simulink model "FOC_For_PMSM"  (R2023b)
settings: Solver=VariableStepAuto  StartTime=0.0  StopTime=1  MaxStep=1e-4  RelTol=1e-3
values from neighbouring files (symbols this model uses):
  B = 11e-5    (= 0.00011)    [FOC_For_PMSM.m]    (also in FOC_For_PMSM_Parameters.m)
  Idref = 0    [FOC_For_PMSM.m]    (also in FOC_For_PMSM_Parameters.m)
  J = 0.47e-4    (= 4.7e-05)    [FOC_For_PMSM.m]    (also in FOC_For_PMSM_Parameters.m)
  Kcq = (2*zeta*wn*L) - Rs    (= 84.52)    [FOC_For_PMSM.m]    (also in FOC_For_PMSM_Parameters.m)
  Kcs = ((2*zeta*wns) - (B/J)) / ((1.5 *(p^2)*flux)/J)    (= 0.00768666666667)    [FOC_For_PMSM.m]    (also in FOC_For_PMSM_Parameters.m)
  Ld = 7e-2    (= 0.07)    [FOC_For_PMSM.m]    (also in FOC_For_PMSM_Parameters.m)
  Lq = 7e-2    (= 0.07)    [FOC_For_PMSM.m]    (also in FOC_For_PMSM_Parameters.m)
  p = 2    [FOC_For_PMSM.m]    (also in FOC_For_PMSM_Parameters.m)
  Rs = 2.98    [FOC_For_PMSM.m]    (also in FOC_For_PMSM_Parameters.m)
  speed_ref = 500    [FOC_For_PMSM.m]    (also in FOC_For_PMSM_Parameters.m)
libraries: slpidlib x3, spsDCVoltageSourceLib x1, spsUniversalBridgeLib x1, spsdq0toabcLib x1, spsPermanentMagnetSynchronousMachineLib x1, spsThreePhaseVIMeasurementLib x1, spspowerguiLib x1
settings Model: Creator=Admin  LastModifiedBy=hkurt
settings SolverCC: ZeroCrossAlgorithm=Adaptive
settings DebuggingCC: MaskedZcDiagnostic=none  IgnoredZcDiagnostic=none

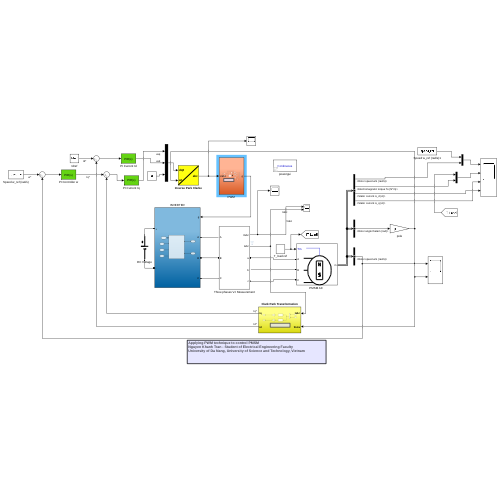
[thumbnail: Simulink's stored preview of the top-level diagram]
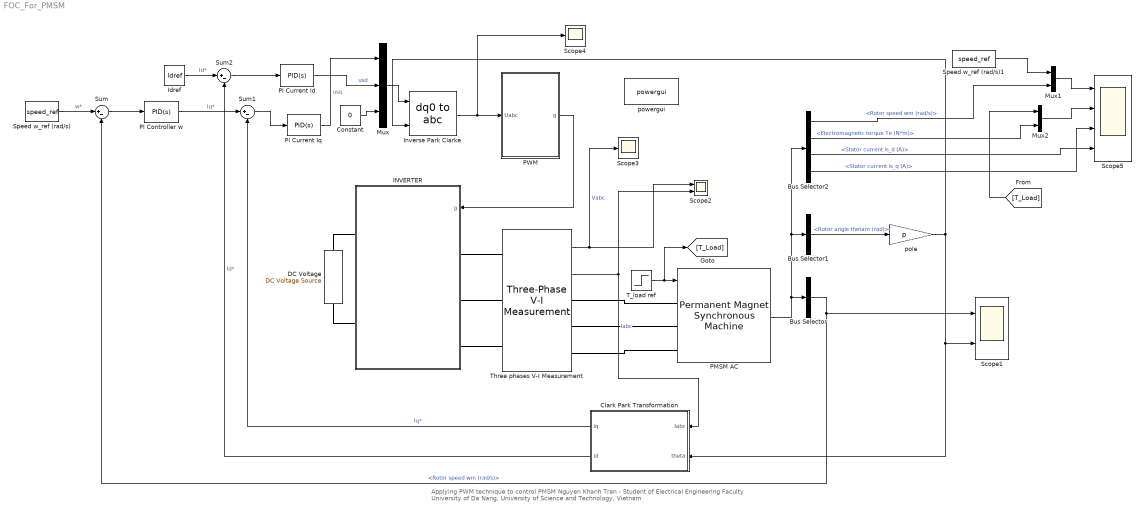
== system FOC_For_PMSM ==
  note: Applying PWM technique to control PMSM
      | Nguyen Khanh Tran - Student of Electrical Engineering Faculty
      | University of Da Nang, University of Science and Technology, Vietnam
  Bus Selector : BusSelector  OutputSignals=Rotor speed wm (rad/s)
  Bus Selector1 : BusSelector  OutputSignals=Rotor angle thetam (rad)
  Bus Selector2 : BusSelector  OutputSignals=Rotor speed wm (rad/s),Electromagnetic torque Te (N*m),Stator current is_d (A),Stator current is_q (A)
  Clark Park Transformation : Subsystem
  Constant : Constant  Value=0
  DC Voltage : spsDCVoltageSourceLib/DC Voltage Source  Amplitude=600  Measurements=None
  INVERTER : Subsystem
  Idref : Constant  Value=Idref
  Inverse Park Clarke : spsdq0toabcLib/dq0 to abc  Alignment=Aligned with phase A axis
  Mux : Mux  Inputs=3
  Mux1 : Mux  Inputs=2
  Mux2 : Mux  Inputs=2
  PI Controller w : slpidlib/PID Controller  Controller=PID  Form=Parallel  TimeDomain=Continuous-time  UseExternalTs=off  SampleTime=-1  IntegratorMethod=Forward Euler  FilterMethod=Forward Euler  ControllerParametersSource=internal  P=Kcs  I=Kcs/0.2001  UseKiTs=off  D=0  N=100  UseFilter=on  TunerSelectOption=Transfer Function Based (PID Tuner App)  InitialConditionSource=internal  InitialConditionForIntegrator=0  InitialConditionForFilter=0  DifferentiatorICPrevScaledInput=0  ExternalReset=none  TrackingMode=off  Kt=1  LimitOutput=off  SatLimitsSource=internal  UpperSaturationLimit=inf  LowerSaturationLimit=-inf  LinearizeAsGain=on  AntiWindupMode=none  Kb=1  LimitIntegrator=off  UpperIntegratorSaturationLimit=inf  LowerIntegratorSaturationLimit=-inf  POutMin=[]  POutMax=[]  IOutMin=[]  IOutMax=[]  DOutMin=[]  DOutMax=[]  NOutMin=[]  NOutMax=[]  SumOutMin=[]  SumOutMax=[]  SaturationOutMin=[]  SaturationOutMax=[]  PParamMin=[]  PParamMax=[]  IParamMin=[]  IParamMax=[]  DParamMin=[]  DParamMax=[]  NParamMin=[]  NParamMax=[]  KbParamMin=[]  KbParamMax=[]  KtParamMin=[]  KtParamMax=[]  KbOutMin=[]  KbOutMax=[]  KtOutMin=[]  KtOutMax=[]  IntegratorOutMin=[]  IntegratorOutMax=[]  FilterOutMin=[]  FilterOutMax=[]  SumI1OutMin=[]  SumI1OutMax=[]  SumI2OutMin=[]  SumI2OutMax=[]  SumI3OutMin=[]  SumI3OutMax=[]  SumI4OutMin=[]  SumI4OutMax=[]  SumDOutMin=[]  SumDOutMax=[]  DifferentiatorOutMin=[]  DifferentiatorOutMax=[]  FilterDiffOutCoefMin=[]  FilterDiffOutCoefMax=[]  ReciprocalOutMin=[]  ReciprocalOutMax=[]  SumDenOutMin=[]  SumDenOutMax=[]  SumNumOutMin=[]  SumNumOutMax=[]  DivideOutMin=[]  DivideOutMax=[]  UdiffTsProdOutMin=[]  UdiffTsProdOutMax=[]  NTsProdOutMin=[]  NTsProdOutMax=[]  UintegralTsProdOutMin=[]  UintegralTsProdOutMax=[]  UngainTsProdOutMin=[]  UngainTsProdOutMax=[]  ClampingZeroOutDataTypeStr=Inherit: Inherit via back propagation  ClampingZeroOutMin=[]  ClampingZeroOutMax=[]  FilterDenConstantOutDataTypeStr=Inherit: Inherit via back propagation  FilterDenConstantOutMin=[]  FilterDenConstantOutMax=[]  PCopyOutDataTypeStr=Inherit: Inherit via back propagation  PCopyOutMin=[]  PCopyOutMax=[]  NCopyOutDataTypeStr=Inherit: Inherit via back propagation  NCopyOutMin=[]  NCopyOutMax=[]  IntegratorContinuousStateAttributes=''  IntegratorStateMustResolveToSignalObject=off  IntegratorRTWStateStorageClass=Auto  FilterContinuousStateAttributes=''  FilterStateMustResolveToSignalObject=off  FilterRTWStateStorageClass=Auto  ParallelPVariant=InternalParameters  IdealPVariant=Disabled  IVariant=InternalParameters  DVariant=InternalParameters  IntegratorVariant=Continuous  SatVariant=Disabled  AWVariant=Passthrough  PCopyVariant=Disabled  TRVariant=Disabled  FdbkBlocksVariant=Forward  IdealPFdbkVariant=Disabled  SatFdbkVariant=Disabled  DerivativeFilterVariant=ContFilter  NVariant=InternalParameters  NCopyVariant=Disabled  FilterICVariant=InternalICsFilter  IntegratorICVariant=InternalICs  ExternalResetVariant=Disabled  TRSumVariant=Passthrough  SumFdbkVariant=Disabled  SumVariant=Sum_PID  TsampFilterVariant=InternalTs  TsampNgainVariant=Passthrough  TsampIntegralVariant=Disabled_SignalSpec  ExternalSaturationOutDataTypeStr=Inherit: Same as second input
  PI Current Id : slpidlib/PID Controller  Controller=PID  Form=Parallel  TimeDomain=Continuous-time  UseExternalTs=off  SampleTime=-1  IntegratorMethod=Forward Euler  FilterMethod=Forward Euler  ControllerParametersSource=internal  P=Kcq  I=Kcq/0.001  UseKiTs=off  D=0  N=100  UseFilter=on  TunerSelectOption=Transfer Function Based (PID Tuner App)  InitialConditionSource=internal  InitialConditionForIntegrator=0  InitialConditionForFilter=0  DifferentiatorICPrevScaledInput=0  ExternalReset=none  TrackingMode=off  Kt=1  LimitOutput=off  SatLimitsSource=internal  UpperSaturationLimit=inf  LowerSaturationLimit=-inf  LinearizeAsGain=on  AntiWindupMode=none  Kb=1  LimitIntegrator=off  UpperIntegratorSaturationLimit=inf  LowerIntegratorSaturationLimit=-inf  POutMin=[]  POutMax=[]  IOutMin=[]  IOutMax=[]  DOutMin=[]  DOutMax=[]  NOutMin=[]  NOutMax=[]  SumOutMin=[]  SumOutMax=[]  SaturationOutMin=[]  SaturationOutMax=[]  PParamMin=[]  PParamMax=[]  IParamMin=[]  IParamMax=[]  DParamMin=[]  DParamMax=[]  NParamMin=[]  NParamMax=[]  KbParamMin=[]  KbParamMax=[]  KtParamMin=[]  KtParamMax=[]  KbOutMin=[]  KbOutMax=[]  KtOutMin=[]  KtOutMax=[]  IntegratorOutMin=[]  IntegratorOutMax=[]  FilterOutMin=[]  FilterOutMax=[]  SumI1OutMin=[]  SumI1OutMax=[]  SumI2OutMin=[]  SumI2OutMax=[]  SumI3OutMin=[]  SumI3OutMax=[]  SumI4OutMin=[]  SumI4OutMax=[]  SumDOutMin=[]  SumDOutMax=[]  DifferentiatorOutMin=[]  DifferentiatorOutMax=[]  FilterDiffOutCoefMin=[]  FilterDiffOutCoefMax=[]  ReciprocalOutMin=[]  ReciprocalOutMax=[]  SumDenOutMin=[]  SumDenOutMax=[]  SumNumOutMin=[]  SumNumOutMax=[]  DivideOutMin=[]  DivideOutMax=[]  UdiffTsProdOutMin=[]  UdiffTsProdOutMax=[]  NTsProdOutMin=[]  NTsProdOutMax=[]  UintegralTsProdOutMin=[]  UintegralTsProdOutMax=[]  UngainTsProdOutMin=[]  UngainTsProdOutMax=[]  ClampingZeroOutDataTypeStr=Inherit: Inherit via back propagation  ClampingZeroOutMin=[]  ClampingZeroOutMax=[]  FilterDenConstantOutDataTypeStr=Inherit: Inherit via back propagation  FilterDenConstantOutMin=[]  FilterDenConstantOutMax=[]  PCopyOutDataTypeStr=Inherit: Inherit via back propagation  PCopyOutMin=[]  PCopyOutMax=[]  NCopyOutDataTypeStr=Inherit: Inherit via back propagation  NCopyOutMin=[]  NCopyOutMax=[]  IntegratorContinuousStateAttributes=''  IntegratorStateMustResolveToSignalObject=off  IntegratorRTWStateStorageClass=Auto  FilterContinuousStateAttributes=''  FilterStateMustResolveToSignalObject=off  FilterRTWStateStorageClass=Auto  ParallelPVariant=InternalParameters  IdealPVariant=Disabled  IVariant=InternalParameters  DVariant=InternalParameters  IntegratorVariant=Continuous  SatVariant=Disabled  AWVariant=Passthrough  PCopyVariant=Disabled  TRVariant=Disabled  FdbkBlocksVariant=Forward  IdealPFdbkVariant=Disabled  SatFdbkVariant=Disabled  DerivativeFilterVariant=ContFilter  NVariant=InternalParameters  NCopyVariant=Disabled  FilterICVariant=InternalICsFilter  IntegratorICVariant=InternalICs  ExternalResetVariant=Disabled  TRSumVariant=Passthrough  SumFdbkVariant=Disabled  SumVariant=Sum_PID  TsampFilterVariant=InternalTs  TsampNgainVariant=Passthrough  TsampIntegralVariant=Disabled_SignalSpec  ExternalSaturationOutDataTypeStr=Inherit: Same as second input
  PI Current Iq : slpidlib/PID Controller  Controller=PID  Form=Parallel  TimeDomain=Continuous-time  UseExternalTs=off  SampleTime=-1  IntegratorMethod=Forward Euler  FilterMethod=Forward Euler  ControllerParametersSource=internal  P=Kcq  I=Kcq/0.001  UseKiTs=off  D=0  N=100  UseFilter=on  TunerSelectOption=Transfer Function Based (PID Tuner App)  InitialConditionSource=internal  InitialConditionForIntegrator=0  InitialConditionForFilter=0  DifferentiatorICPrevScaledInput=0  ExternalReset=none  TrackingMode=off  Kt=1  LimitOutput=off  SatLimitsSource=internal  UpperSaturationLimit=inf  LowerSaturationLimit=-inf  LinearizeAsGain=on  AntiWindupMode=none  Kb=1  LimitIntegrator=off  UpperIntegratorSaturationLimit=inf  LowerIntegratorSaturationLimit=-inf  POutMin=[]  POutMax=[]  IOutMin=[]  IOutMax=[]  DOutMin=[]  DOutMax=[]  NOutMin=[]  NOutMax=[]  SumOutMin=[]  SumOutMax=[]  SaturationOutMin=[]  SaturationOutMax=[]  PParamMin=[]  PParamMax=[]  IParamMin=[]  IParamMax=[]  DParamMin=[]  DParamMax=[]  NParamMin=[]  NParamMax=[]  KbParamMin=[]  KbParamMax=[]  KtParamMin=[]  KtParamMax=[]  KbOutMin=[]  KbOutMax=[]  KtOutMin=[]  KtOutMax=[]  IntegratorOutMin=[]  IntegratorOutMax=[]  FilterOutMin=[]  FilterOutMax=[]  SumI1OutMin=[]  SumI1OutMax=[]  SumI2OutMin=[]  SumI2OutMax=[]  SumI3OutMin=[]  SumI3OutMax=[]  SumI4OutMin=[]  SumI4OutMax=[]  SumDOutMin=[]  SumDOutMax=[]  DifferentiatorOutMin=[]  DifferentiatorOutMax=[]  FilterDiffOutCoefMin=[]  FilterDiffOutCoefMax=[]  ReciprocalOutMin=[]  ReciprocalOutMax=[]  SumDenOutMin=[]  SumDenOutMax=[]  SumNumOutMin=[]  SumNumOutMax=[]  DivideOutMin=[]  DivideOutMax=[]  UdiffTsProdOutMin=[]  UdiffTsProdOutMax=[]  NTsProdOutMin=[]  NTsProdOutMax=[]  UintegralTsProdOutMin=[]  UintegralTsProdOutMax=[]  UngainTsProdOutMin=[]  UngainTsProdOutMax=[]  ClampingZeroOutDataTypeStr=Inherit: Inherit via back propagation  ClampingZeroOutMin=[]  ClampingZeroOutMax=[]  FilterDenConstantOutDataTypeStr=Inherit: Inherit via back propagation  FilterDenConstantOutMin=[]  FilterDenConstantOutMax=[]  PCopyOutDataTypeStr=Inherit: Inherit via back propagation  PCopyOutMin=[]  PCopyOutMax=[]  NCopyOutDataTypeStr=Inherit: Inherit via back propagation  NCopyOutMin=[]  NCopyOutMax=[]  IntegratorContinuousStateAttributes=''  IntegratorStateMustResolveToSignalObject=off  IntegratorRTWStateStorageClass=Auto  FilterContinuousStateAttributes=''  FilterStateMustResolveToSignalObject=off  FilterRTWStateStorageClass=Auto  ParallelPVariant=InternalParameters  IdealPVariant=Disabled  IVariant=InternalParameters  DVariant=InternalParameters  IntegratorVariant=Continuous  SatVariant=Disabled  AWVariant=Passthrough  PCopyVariant=Disabled  TRVariant=Disabled  FdbkBlocksVariant=Forward  IdealPFdbkVariant=Disabled  SatFdbkVariant=Disabled  DerivativeFilterVariant=ContFilter  NVariant=InternalParameters  NCopyVariant=Disabled  FilterICVariant=InternalICsFilter  IntegratorICVariant=InternalICs  ExternalResetVariant=Disabled  TRSumVariant=Passthrough  SumFdbkVariant=Disabled  SumVariant=Sum_PID  TsampFilterVariant=InternalTs  TsampNgainVariant=Passthrough  TsampIntegralVariant=Disabled_SignalSpec  ExternalSaturationOutDataTypeStr=Inherit: Same as second input
  "PMSM AC  " : spsPermanentMagnetSynchronousMachineLib/Permanent Magnet Synchronous Machine  NbPhases=3  FluxDistribution=Sinusoidal  RotorType=Salient-pole  MechanicalLoad=Torque Tm  PresetModel=No  ShowDetailedParameters=on  MeasurementBus=off  Resistance=Rs  Inductance=8.5e-3  dqInductances=[Ld, Lq]  La=0.000395  MachineConstant=Flux linkage established by magnets (V.s)  Flux=flux  VoltageCst=45.345  TorqueCst=0.375  Flat=120  Mechanical=[J B p 0]  PolePairs=4  InitialConditions=[0,0, 0,0]  InitialConditions5ph=[0 0 0 0 0 0]  RefAngle=90 degrees behind phase A axis (modified Park)  IterativeDiscreteModel=Trapezoidal non iterative  TsBlock=-1  TsPowergui=0
  "PWM " : Subsystem
  Scope1 : Scope  NumInputPorts=2
  Scope2 : Scope  NumInputPorts=2
  Scope3 : Scope
  Scope4 : Scope
  Scope5 : Scope  NumInputPorts=4
  Speed w_ref (rad/s) : Constant  Value=speed_ref
  Speed w_ref (rad/s)1 : Constant  Value=speed_ref
  Sum : Sum  Inputs=|+-
  Sum1 : Sum  Inputs=|+-
  Sum2 : Sum  Inputs=|+-
  T_load ref : Step  Time=0.3  SampleTime=0
  Three phases V-I Measurement : spsThreePhaseVIMeasurementLib/Three-Phase V-I Measurement  VoltageMeasurement=phase-to-phase  SetLabelV=off  LabelV=Vabc  Vpu=off  VpuLL=off  CurrentMeasurement=yes  SetLabelI=off  LabelI=Iabc  Ipu=off  Pbase=100e6  Vbase=500e3  OutputType=Complex  PhasorSimulation=off  PSBequivalent=0
  pole : Gain  Gain=p
  powergui : spspowerguiLib/powergui  Priority=1  SimulationMode=Continuous  SampleTime=50e-6  frequency=60  Iterations=50  frequencyindice=0  Pbase=100e6  ErrMax=1e-4  UnitsV=kV  UnitsW=MW  buscounter=0  FunctionMessages=off  echomessages=off  EnableUseOfTLC=off  CurrentSourceSwitches=off  DisableSnubberDevices=off  DisableRonSwitches=off  DisableVfSwitches=off  DisplayEquations=off  AutomaticDiscreteSolvers=off  SolverType=Tustin/Backward Euler (TBE)  Interpol=off  ExternalGateDelay=off  methode=off  Ts=100  x0status=blocks  SPID=on  SwTol=0  HookPort=off  NonlinearTolerance=1e-4  nMaxIteration=100  ContinueOnMaxIteration=off  RestoreLinks=warning  ResistiveCurrentMeasurement=off  Frange=[0:2:500]  Ylog=off  Xlog=on  ShowGrid=off  save=off  variable=ZData  structure=0  ZoomFFT=off  StartTime=0.0  cycles=1  DisplayStyle=1  fundamental=60  FreqAxis=off  MaxFrequency=1000  frequencyindicesteady=1  RmsSteady=1  display=off
  wires:
  Sum/1 -> PI Controller w/1
  Speed w_ref (rad/s)/1 -> Sum/1  "w*"
  "PMSM AC  "/1 -> Bus Selector2/1, Bus Selector1/1, Bus Selector/1
  Bus Selector1/1 -> pole/1  "<Rotor angle thetam (rad)>"
  Bus Selector2/2 -> Mux2/2  "<Electromagnetic torque Te (N*m)>"
  Bus Selector2/3 -> Scope5/4  "<Stator current is_d (A)>"
  Bus Selector2/4 -> Scope5/3  "<Stator current is_q (A)>"
  Three phases V-I Measurement/1 -> Scope3/1, Scope2/1  "Vabc"
  Sum1/1 -> PI Current Iq/1
  Sum2/1 -> PI Current Id/1
  Idref/1 -> Sum2/1  "Id*"
  PI Controller w/1 -> Sum1/1  "Iq*"
  "PWM "/1(g) -> INVERTER/1(g)
  Three phases V-I Measurement/2 -> Clark Park Transformation/1(Iabc), Scope2/2  "Iabc"
  Mux/1 -> Inverse Park Clarke/1
  Inverse Park Clarke/1 -> Scope4/1, "PWM "/1(Uabc)
  Constant/1 -> Mux/3
  pole/1 -> Clark Park Transformation/2(theta), Scope1/2, Inverse Park Clarke/2
  PI Current Id/1 -> Mux/2  "usd"
  PI Current Iq/1 -> Mux/1  "usq"
  Bus Selector/1 -> Sum/2, Scope1/1  "<Rotor speed wm (rad/s)>"
  Clark Park Transformation/1(iq) -> Sum1/2  "Iq*"
  Clark Park Transformation/2(id) -> Sum2/2  "Id*"
  [T_Load] -> Mux2/1
  Speed w_ref (rad/s)1/1 -> Mux1/1
  Mux1/1 -> Scope5/1
  Mux2/1 -> Scope5/2
  Bus Selector2/1 -> Mux1/2  "<Rotor speed wm (rad/s)>"
  T_load ref/1 -> [T_Load], "PMSM AC  "/1
  connections:
  INVERTER/LConn1 -- Three phases V-I Measurement/LConn1
  INVERTER/LConn2 -- Three phases V-I Measurement/LConn2
  INVERTER/LConn3 -- Three phases V-I Measurement/LConn3
  Three phases V-I Measurement/RConn1 -- "PMSM AC  "/LConn1
  Three phases V-I Measurement/RConn2 -- "PMSM AC  "/LConn2
  Three phases V-I Measurement/RConn3 -- "PMSM AC  "/LConn3
  DC Voltage/RConn1 -- INVERTER/RConn1
  INVERTER/RConn2 -- DC Voltage/LConn1

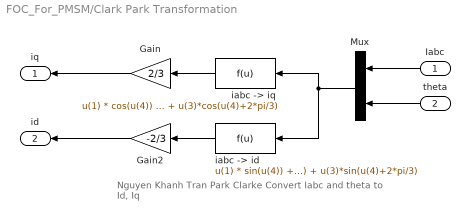
== system FOC_For_PMSM/Clark Park Transformation ==
  note: Nguyen Khanh Tran
      | Park Clarke
      | Convert Iabc and theta to Id, Iq
  Iabc : Inport
  theta : Inport  Port=2
  Gain : Gain  Gain=2/3
  Gain2 : Gain  Gain=-2/3
  Mux : Mux  Inputs=2
  "iabc -> id" : Fcn  Expr=u(1) * sin(u(4)) + u(2) *sin(u(4) - 2*pi/3) + u(3)*sin(u(4)+2*pi/3)
  "iabc -> iq" : Fcn  Expr=u(1) * cos(u(4)) + u(2) *cos(u(4) - 2*pi/3) + u(3)*cos(u(4)+2*pi/3)
  iq : Outport
  id : Outport  Port=2
  wires:
  Mux/1 -> "iabc -> iq"/1, "iabc -> id"/1
  "iabc -> id"/1 -> Gain2/1
  Gain2/1 -> id/1
  "iabc -> iq"/1 -> Gain/1
  Gain/1 -> iq/1
  Iabc/1 -> Mux/1
  theta/1 -> Mux/2

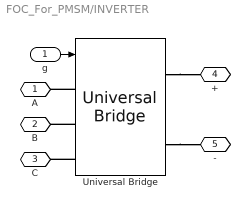
== system FOC_For_PMSM/INVERTER ==
  g : Inport
  Universal Bridge : spsUniversalBridgeLib/Universal Bridge  Arms=3  SnubberResistance=1e5  SnubberCapacitance=inf  Device=IGBT / Diodes  Ron=1e-3  Lon=0  ForwardVoltages="[  0  0  ]"  ForwardVoltage=0  GTOparameters=[ 10e-6 , 20e-6 ]  IGBTparameters=[ 1e-6 , 2e-6 ]  Measurements=None  Measurements_2=None  converterType=Rectifier
  A : PMIOPort  Side=Left
  B : PMIOPort  Port=2  Side=Left
  C : PMIOPort  Port=3  Side=Left
  + : PMIOPort  Port=4  Side=Right
  - : PMIOPort  Port=5  Side=Right
  wires:
  g/1 -> Universal Bridge/1
  connections:
  Universal Bridge/LConn1 -- A/RConn1
  Universal Bridge/RConn1 -- +/RConn1
  Universal Bridge/RConn2 -- -/RConn1
  Universal Bridge/LConn3 -- C/RConn1
  Universal Bridge/LConn2 -- B/RConn1

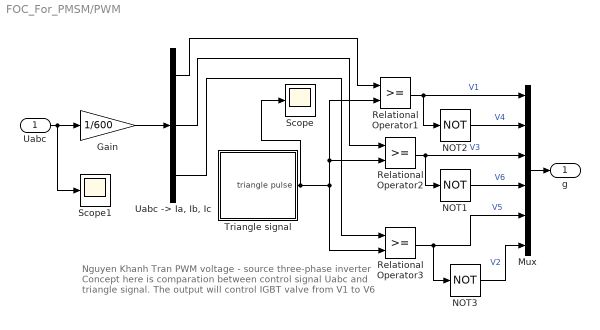
== system FOC_For_PMSM/PWM  ==
  note: Nguyen Khanh Tran
      | PWM voltage - source three-phase inverter
      | Concept here is comparation between
      | control signal Uabc and triangle signal.
      | The output will control IGBT valve from V1 to V6
  Uabc : Inport
  Gain : Gain  Gain=1/600
  Mux : Mux  Inputs=6
  NOT1 : Logic  Operator=NOT  IconShape=distinctive  AllPortsSameDT=off  OutDataTypeStr=boolean
  NOT2 : Logic  Operator=NOT  IconShape=distinctive  AllPortsSameDT=off  OutDataTypeStr=boolean
  NOT3 : Logic  Operator=NOT  IconShape=distinctive  AllPortsSameDT=off  OutDataTypeStr=boolean
  Relational Operator1 : RelationalOperator  OutDataTypeStr=boolean  RndMeth=Simplest  InputSameDT=off
  Relational Operator2 : RelationalOperator  OutDataTypeStr=boolean  RndMeth=Simplest  InputSameDT=off
  Relational Operator3 : RelationalOperator  OutDataTypeStr=boolean  RndMeth=Simplest  InputSameDT=off
  Scope : Scope
  Scope1 : Scope
  "Triangle signal " : Subsystem
  "Uabc -> Ia, Ib, Ic " : Demux  Outputs=3
  g : Outport
  wires:
  NOT1/1 -> Mux/4  "V6"
  "Uabc -> Ia, Ib, Ic "/2 -> Relational Operator2/1
  "Uabc -> Ia, Ib, Ic "/1 -> Relational Operator1/1
  "Uabc -> Ia, Ib, Ic "/3 -> Relational Operator3/1
  Relational Operator2/1 -> NOT1/1, Mux/3  "V3"
  Relational Operator1/1 -> NOT2/1, Mux/1  "V1"
  "Triangle signal "/1(triangle pulse) -> Relational Operator2/2, Relational Operator1/2, Relational Operator3/2, Scope/1
  Relational Operator3/1 -> NOT3/1, Mux/5  "V5"
  NOT3/1 -> Mux/6  "V2"
  NOT2/1 -> Mux/2  "V4"
  Mux/1 -> g/1
  Uabc/1 -> Scope1/1, Gain/1
  Gain/1 -> "Uabc -> Ia, Ib, Ic "/1

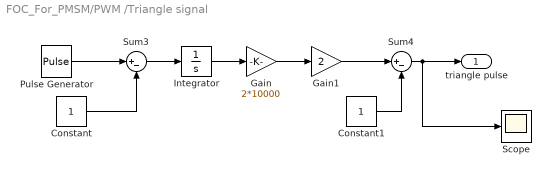
== system FOC_For_PMSM/PWM /Triangle signal  ==
  Constant : Constant
  Constant1 : Constant
  Gain : Gain  Gain=2*10000
  Gain1 : Gain  Gain=2
  Integrator : Integrator
  Pulse Generator : DiscretePulseGenerator  PulseType=Time based  Amplitude=2  Period=1/10000  PulseWidth=50
  Scope : Scope
  Sum3 : Sum  Inputs=|+-
  Sum4 : Sum  Inputs=|+-
  triangle pulse : Outport
  wires:
  Integrator/1 -> Gain/1
  Gain/1 -> Gain1/1
  Constant1/1 -> Sum4/2
  Gain1/1 -> Sum4/1
  Pulse Generator/1 -> Sum3/1
  Sum3/1 -> Integrator/1
  Constant/1 -> Sum3/2
  Sum4/1 -> Scope/1, triangle pulse/1
